simulink model "Problem6"  (R2020b)
settings: Solver=VariableStepAuto  StartTime=0.0  StopTime=10.0  RelTol=1e-3
settings Model: Creator=Acer  LastModifiedBy=Acer

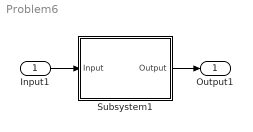
== system Problem6 ==
  Input1 : Inport
  Subsystem1 : Subsystem
  Output1 : Outport
  wires:
  Subsystem1/1(Output) -> Output1/1
  Input1/1 -> Subsystem1/1(Input)

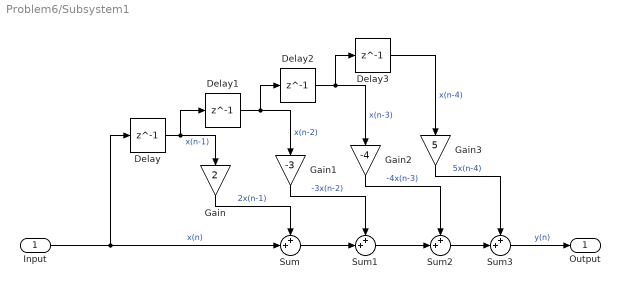
== system Problem6/Subsystem1 ==
  Input : Inport
  Delay{,1..3} (4 alike) : Delay  DelayLength=1
  Gain : Gain  Gain=2
  Gain1 : Gain  Gain=-3
  Gain2 : Gain  Gain=-4
  Gain3 : Gain  Gain=5
  Sum{,1..3} (4 alike) : Sum  Inputs=++|
  Output : Outport
  wires:
  Gain1/1 -> Sum1/1  "-3x(n-2)"
  Sum1/1 -> Sum2/2
  Gain3/1 -> Sum3/1  "5x(n-4)"
  Gain2/1 -> Sum2/1  "-4x(n-3)"
  Gain/1 -> Sum/1  "2x(n-1)"
  Delay3/1 -> Gain3/1  "x(n-4)"
  Sum2/1 -> Sum3/2
  Delay2/1 -> Gain2/1, Delay3/1  "x(n-3)"
  Sum3/1 -> Output/1  "y(n)"
  Sum/1 -> Sum1/2
  Delay/1 -> Gain/1, Delay1/1  "x(n-1)"
  Input/1 -> Sum/2, Delay/1  "x(n)"
  Delay1/1 -> Gain1/1, Delay2/1  "x(n-2)"
